simulink model "FOC_HF_G474"  (R2020b)
settings: Solver=FixedStepDiscrete  StartTime=0.0  StopTime=10  FixedStep=TsBSP  RelTol=1e-3
values from neighbouring files (symbols this model uses):
  BandwidthCurrentPI = 314.15926535897933    [G474_FOC_HF.sldd]
  Ld = 4.9E-5    [G474_FOC_HF.sldd]    (also in Hall_HFI_FOC_Data.sldd = 0.0004
  Ld_MODEL = 4.9E-5    [G474_FOC_HF.sldd]
  Lq = 4.9E-5    [G474_FOC_HF.sldd]    (also in Hall_HFI_FOC_Data.sldd = 0.00045
  Lq_MODEL = 4.9E-5    [G474_FOC_HF.sldd]
  MaxVoltage = 5.0    [G474_FOC_HF.sldd]
  PolePairs = 5.0    [G474_FOC_HF.sldd]
  PolePairs_MODEL = 5.0    [G474_FOC_HF.sldd]
  PWMHalfPeriod = 4199.0    [G474_FOC_HF.sldd]
  Rs = 0.082    [G474_FOC_HF.sldd]
  TsBSP = 2.0E-5    [G474_FOC_HF.sldd]
  TsFOC = 0.0001    [G474_FOC_HF.sldd]
  TsFOC_MODEL = 0.0001    [G474_FOC_HF.sldd]
undefined symbols (not defined in the file or in its folder): sigbuilder_block
libraries: pid_lib x4, mcbplantlib x1, autolibpmsminterior x1
(part 1 of 2)
PreSaveFcn:
  | cd(fileparts(which(bdroot)));
settings Model: DataDictionary=G474_FOC_HF.sldd  PacingRate=1000  Creator=beau_  LastModifiedBy=beau_
settings DataIOCC: SaveOutput=off  DSMLogging=off  SaveTime=off  ReturnWorkspaceOutputs=off
settings OptimizationCC: DefaultParameterBehavior=Inlined  EnhancedBackFolding=on  PassReuseOutputArgsAs=Individual arguments  ZeroExternalMemoryAtStartup=off  OptimizeBlockOrder=speed  DifferentSizesBufferReuse=on  OptimizationCustomize=off  EfficientTunableParamExpr=on
settings DebuggingCC: SignalRangeChecking=warning  ParameterPrecisionLossMsg=none  ParameterTunabilityLossMsg=error
settings HardwareCC: ProdBitPerPointer=32  ProdBitPerSizeT=32  ProdBitPerPtrDiffT=32  ProdLargestAtomicInteger=Long  ProdLargestAtomicFloat=Double  ProdWordSize=32  ProdHWDeviceType=ARM Compatible->ARM Cortex-M
settings SFSimCC: SimParseCustomCode=off  MATLABDynamicMemAlloc=off
settings RTWCC: Description=Embedded Coder  SystemTargetFile=ert.tlc  GenCodeOnly=on  TemplateMakefile=ert_default_tmf  RTWUseSimCustomCode=on
settings CodeAppCC: ForceParamTrailComments=on  GenerateComments=off  IgnoreCustomStorageClasses=off  OperatorAnnotations=on  SimulinkDataObjDesc=on  SFDataObjDesc=on  InsertBlockDesc=on
settings ERTTargetCC: TargetLangStandard=C99 (ISO)  CodeReplacementLibrary=ARM Cortex-M  GenerateSampleERTMain=on  SupportAbsoluteTime=off  SupportNonFinite=off  SupportComplex=off  InlinedParameterPlacement=NonHierarchical  ERTCustomFileTemplate=example_file_process.tlc

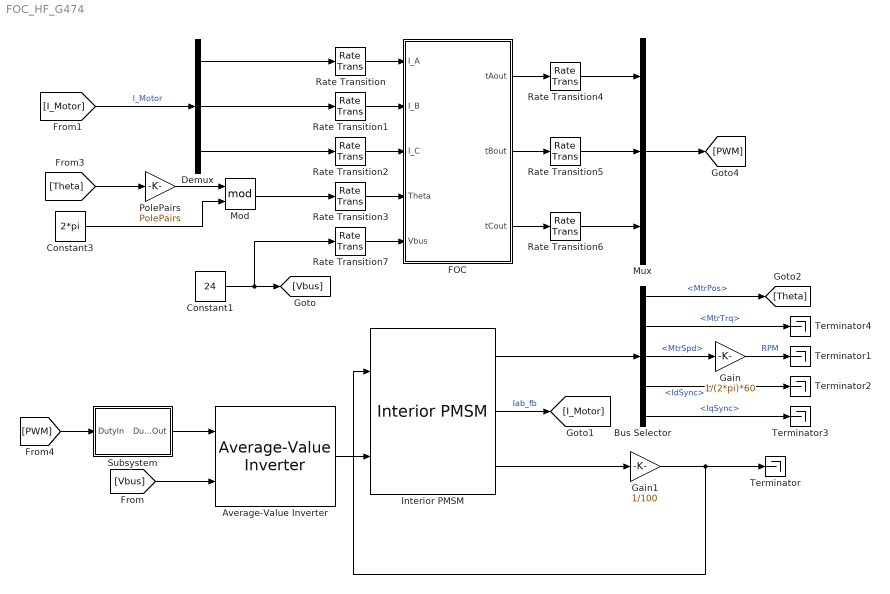
== system FOC_HF_G474 ==
  Average-Value Inverter : mcbplantlib/Average-Value Inverter
  Bus Selector : BusSelector  OutputSignals=MtrPos,MtrTrq,MtrSpd,IdSync,IqSync
  Constant1 : Constant  Value=24  SampleTime=TsBSP
  Constant3 : Constant  Value=2*pi  SampleTime=TsBSP
  Demux : Demux  Outputs=3
  FOC : Subsystem  SystemSampleTime=TsFOC
  Gain : Gain  Gain=1/(2*pi)*60
  Gain1 : Gain  Gain=1/100
  Interior PMSM : autolibpmsminterior/Interior PMSM  port_config=Torque  sim_type=Discrete  Ts=TsBSP  P=PolePairs_MODEL  Rs=Rs_MODEL  Ldq=[Ld_MODEL Lq_MODEL]  KConstText=Permanent flux linkage constant (lambda_pm):  lambda_pm=Flux_MODEL  Ke=159.9771  mechanical=[2.8e-4,1e-5,0.01]  idq0=[0 0]  theta_init=pi/4/PolePairs_MODEL  omega_init=0  KConst=Flux_MODEL  lambda_pm_calc=Flux_MODEL  Kt=0.07  RefBlkName='autolibpmsminterior/Interior PMSM'  aMode=5
      settings: SourceProductBaseCode=PW,MT,UV,VE,VP
  Mod : Math  Operator=mod  SaturateOnIntegerOverflow=on
  Mux : Mux  Inputs=3
  PolePairs : Gain  Gain=PolePairs
  Rate Transition{,1..3,7} (5 alike) : RateTransition
  Rate Transition4 : RateTransition  OutPortSampleTime=TsBSP
  Rate Transition5 : RateTransition  OutPortSampleTime=TsBSP
  Rate Transition6 : RateTransition  OutPortSampleTime=TsBSP
  Subsystem : Subsystem
  Terminator{,1..4} (5 alike) : Terminator
  wires:
  Average-Value Inverter/1 -> Interior PMSM/2
  Rate Transition4/1 -> Mux/1
  Interior PMSM/2 -> [I_Motor]  "Iab_fb"
  Rate Transition7/1 -> FOC/5(Vbus)
  Interior PMSM/3 -> Gain1/1
  Bus Selector/5 -> Terminator3/1  "<IqSync>"
  Bus Selector/4 -> Terminator2/1  "<IdSync>"
  [Vbus] -> Average-Value Inverter/2
  Mux/1 -> [PWM]
  Rate Transition2/1 -> FOC/3(I_C)
  Mod/1 -> Rate Transition3/1
  PolePairs/1 -> Mod/1
  Subsystem/1(DutyOut) -> Average-Value Inverter/1
  Constant1/1 -> Rate Transition7/1, [Vbus]
  Rate Transition3/1 -> FOC/4(Theta)
  Demux/3 -> Rate Transition2/1
  Rate Transition/1 -> FOC/1(I_A)
  Demux/1 -> Rate Transition/1
  Gain1/1 -> Interior PMSM/1, Terminator/1
  Rate Transition5/1 -> Mux/2
  Interior PMSM/1 -> Bus Selector/1
  Rate Transition6/1 -> Mux/3
  Bus Selector/1 -> [Theta]  "<MtrPos>"
  FOC/2(tBout) -> Rate Transition5/1
  [Theta] -> PolePairs/1
  FOC/3(tCout) -> Rate Transition6/1
  FOC/1(tAout) -> Rate Transition4/1
  Demux/2 -> Rate Transition1/1
  Bus Selector/3 -> Gain/1  "<MtrSpd>"
  Constant3/1 -> Mod/2
  Rate Transition1/1 -> FOC/2(I_B)
  [PWM] -> Subsystem/1(DutyIn)
  [I_Motor] -> Demux/1  "I_Motor"
  Gain/1 -> Terminator1/1  "RPM"
  Bus Selector/2 -> Terminator4/1  "<MtrTrq>"

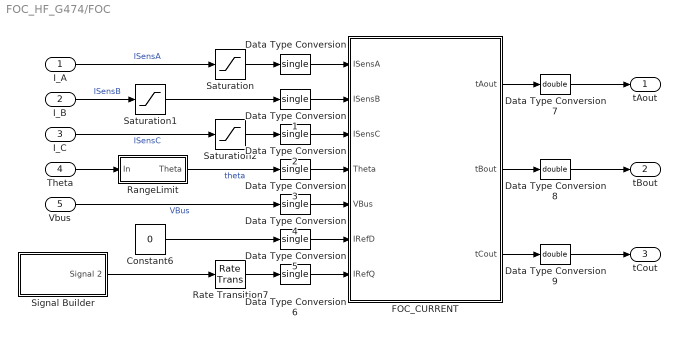
== system FOC_HF_G474/FOC ==
  I_A : Inport
  I_B : Inport  Port=2
  I_C : Inport  Port=3
  Theta : Inport  Port=4  OutMin=-2*pi  OutMax=2*pi
  Vbus : Inport  Port=5
  Constant6 : Constant  Value=0  SampleTime=-1
  Data Type Conversion{,1..6} (7 alike) : DataTypeConversion  OutDataTypeStr=single
  Data Type Conversion7 : DataTypeConversion  OutDataTypeStr=double
  Data Type Conversion8 : DataTypeConversion  OutDataTypeStr=double
  Data Type Conversion9 : DataTypeConversion  OutDataTypeStr=double
  FOC_CURRENT : Subsystem  TreatAsAtomicUnit=on  SystemSampleTime=TsFOC_MODEL
  RangeLimit : Subsystem
  Rate Transition7 : RateTransition
  Saturation : Saturate  UpperLimit=100  LowerLimit=-100
  Saturation1 : Saturate  UpperLimit=100  LowerLimit=-100
  Saturation2 : Saturate  UpperLimit=100  LowerLimit=-100
  Signal Builder : Subsystem  Tag=STV Subsys  LoadFcn=sigbuilder_block('load');  StartFcn=sigbuilder_block('start');  StopFcn=sigbuilder_block('stop');  ClipboardFcn=sigbuilder_block('clipboard');  mask(Sigbuilder block){tuvar=[0:10]}
      mask help: Simulink:masks:SigbuilderBlock_MD
      mask init:
      | if ~strcmp(get_param(bdroot(gcbh),'SimulationStatus'),'stopped') tuvar = sigbuilder_block('maskInit'); end
      settings: CopyFcn=sigbuilder_block('copy');  DeleteFcn=sigbuilder_block('delete');  ModelCloseFcn=sigbuilder_block('modelClose');  PreSaveFcn=sigbuilder_block('preSave');  PauseFcn=sigbuilder_block('pause');  ContinueFcn=sigbuilder_block('continue');  NameChangeFcn=sigbuilder_block('namechange');  OpenFcn=sigbuilder_block('open',[50.25 51 1141.5 581.25 ]);  CloseFcn=sigbuilder_block('close');
      mask Display: plot(0, 0, 100, 100,[2, 2, 32, 32, 2], [68, 8, 8, 68, 68],[32, 2], [38, 38], [32, 19, 2],[53, 60, 44], [32, 17, 17, 2],[16, 16, 31, 31]);txt = getActiveGroup(gcbh);text(2, 100, txt,'verticalAlignment', 'top');
  tAout : Outport
  tBout : Outport  Port=2
  tCout : Outport  Port=3
  wires:
  I_A/1 -> Saturation/1  "ISensA"
  I_C/1 -> Saturation2/1  "ISensC"
  Vbus/1 -> Data Type Conversion4/1  "VBus"
  I_B/1 -> Saturation1/1  "ISensB"
  Constant6/1 -> Data Type Conversion5/1
  Theta/1 -> RangeLimit/1(In)
  FOC_CURRENT/3(tCout) -> Data Type Conversion9/1
  FOC_CURRENT/1(tAout) -> Data Type Conversion7/1
  FOC_CURRENT/2(tBout) -> Data Type Conversion8/1
  Saturation/1 -> Data Type Conversion/1
  Saturation1/1 -> Data Type Conversion1/1
  Saturation2/1 -> Data Type Conversion2/1
  RangeLimit/1(Theta) -> Data Type Conversion3/1  "theta"
  Signal Builder/1(Signal 2) -> Rate Transition7/1
  Rate Transition7/1 -> Data Type Conversion6/1
  Data Type Conversion/1 -> FOC_CURRENT/1(ISensA)
  Data Type Conversion1/1 -> FOC_CURRENT/2(ISensB)
  Data Type Conversion2/1 -> FOC_CURRENT/3(ISensC)
  Data Type Conversion3/1 -> FOC_CURRENT/4(Theta)
  Data Type Conversion4/1 -> FOC_CURRENT/5(VBus)
  Data Type Conversion5/1 -> FOC_CURRENT/6(IRefD)
  Data Type Conversion6/1 -> FOC_CURRENT/7(IRefQ)
  Data Type Conversion7/1 -> tAout/1
  Data Type Conversion8/1 -> tBout/1
  Data Type Conversion9/1 -> tCout/1

== system FOC_HF_G474/Subsystem ==
  DutyIn : Inport
  Constant : Constant  Value=0.5  SampleTime=TsBSP
  Gain : Gain  Gain=1/PWMHalfPeriod  ParamDataTypeStr=single
  Gain1 : Gain  Gain=-1
  Sum : Sum  Inputs=|+-
  Sum1 : Sum  Inputs=|++
  DutyOut : Outport
  wires:
  Sum/1 -> Gain1/1
  Constant/1 -> Sum1/2, Sum/2
  DutyIn/1 -> Gain/1
  Gain1/1 -> Sum1/1
  Sum1/1 -> DutyOut/1
  Gain/1 -> Sum/1

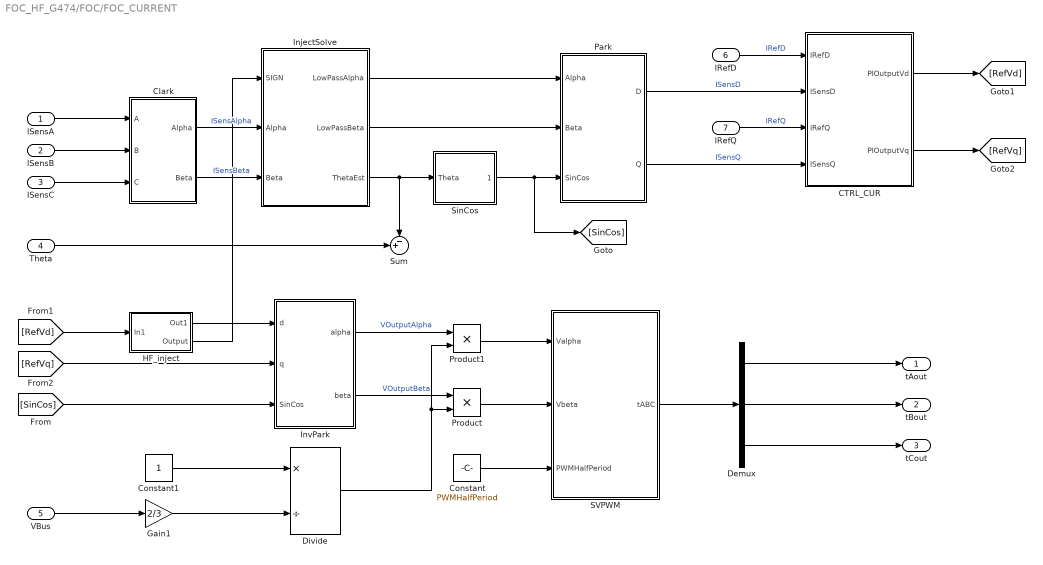
== system FOC_HF_G474/FOC/FOC_CURRENT ==
  ISensA : Inport  OutMin=-100  OutMax=100
  ISensB : Inport  Port=2  OutMin=-100  OutMax=100
  ISensC : Inport  Port=3  OutMin=-100  OutMax=100
  Theta : Inport  Port=4  OutMin=-2*pi  OutMax=2*pi
  VBus : Inport  Port=5  OutMin=0  OutMax=500
  IRefD : Inport  Port=6  OutMin=-50  OutMax=50
  IRefQ : Inport  Port=7  OutMin=-50  OutMax=50
  CTRL_CUR : Subsystem  TreatAsAtomicUnit=on
  Clark : Subsystem  TreatAsAtomicUnit=on
      settings: RTWSystemCode=Inline  RTWFcnNameOpts=Use subsystem name
      mask Display:
      | port_label('input',1,'a','texmode','on');
      | port_label('input',2,'b','texmode','on');
      | port_label('input',3,'c','texmode','on');
      | 
      | port_label('output',1,'\alpha','texmode','on');
      | port_label('output',2,'\beta','texmode','on');
      | 
      | fprintf('Clark');
  Constant : Constant  Value=PWMHalfPeriod  OutDataTypeStr=single  SampleTime=-1
  Constant1 : Constant  OutDataTypeStr=single  SampleTime=-1
  Demux : Demux  Outputs=3
  Divide : Product  Inputs=*/
  Gain1 : Gain  Gain=2/3
  HF_inject : Subsystem
  InjectSolve : Subsystem  TreatAsAtomicUnit=on
  InvPark : Subsystem  TreatAsAtomicUnit=on
      settings: RTWFcnNameOpts=Use subsystem name
      mask Display:
      | port_label('input',1,'d','texmode','on');
      | port_label('input',2,'q','texmode','on');
      | port_label('input',3,'\theta','texmode','on');
      | 
      | port_label('output',1,'\alpha','texmode','on');
      | port_label('output',2,'\beta','texmode','on');
      | 
      | fprintf('Inverse\nPark')
  Park : Subsystem  TreatAsAtomicUnit=on
      settings: RTWFcnNameOpts=Use subsystem name
      mask Display:
      | port_label('input',1,'\alpha','texmode','on');
      | port_label('input',2, '\beta','texmode','on');
      | port_label('input',3, 'sin\thetacos\theta','texmode','on');
      | 
      | port_label('output',1,'d','texmode','on');
      | port_label('output',2,'q','texmode','on');
      | fprintf('Park');
  Product : Product
  Product1 : Product
  SVPWM : Subsystem  TreatAsAtomicUnit=on
  SinCos : Subsystem
  Sum : Sum  Inputs=-+|
  tAout : Outport
  tBout : Outport  Port=2
  tCout : Outport  Port=3
  wires:
  Constant1/1 -> Divide/1
  CTRL_CUR/2(PIOutputVq) -> [RefVq]
  [RefVq] -> InvPark/2(q)
  InvPark/1(alpha) -> Product1/1  "VOutputAlpha"
  ISensB/1 -> Clark/2(B)
  IRefQ/1 -> CTRL_CUR/3(IRefQ)  "IRefQ"
  Divide/1 -> Product1/2, Product/2
  Product/1 -> SVPWM/2(Vbeta)
  Park/2(Q) -> CTRL_CUR/4(ISensQ)  "ISensQ"
  Gain1/1 -> Divide/2
  [SinCos] -> InvPark/3(SinCos)
  IRefD/1 -> CTRL_CUR/1(IRefD)  "IRefD"
  InvPark/2(beta) -> Product/1  "VOutputBeta"
  [RefVd] -> HF_inject/1(In1)
  Constant/1 -> SVPWM/3(PWMHalfPeriod)
  Park/1(D) -> CTRL_CUR/2(ISensD)  "ISensD"
  VBus/1 -> Gain1/1
  CTRL_CUR/1(PIOutputVd) -> [RefVd]
  SinCos/1(SinCos) -> [SinCos], Park/3(SinCos)
  ISensC/1 -> Clark/3(C)
  ISensA/1 -> Clark/1(A)
  Product1/1 -> SVPWM/1(Valpha)
  SVPWM/1(tABC) -> Demux/1
  Demux/1 -> tAout/1
  Demux/2 -> tBout/1
  Demux/3 -> tCout/1
  HF_inject/1(Out1) -> InvPark/1(d)
  Clark/1(Alpha) -> InjectSolve/2(Alpha)  "ISensAlpha"
  Clark/2(Beta) -> InjectSolve/3(Beta)  "ISensBeta"
  HF_inject/2(Output) -> InjectSolve/1(SIGN)
  InjectSolve/1(LowPassAlpha) -> Park/1(Alpha)
  InjectSolve/2(LowPassBeta) -> Park/2(Beta)
  InjectSolve/3(ThetaEst) -> Sum/1, SinCos/1(Theta)
  Theta/1 -> Sum/2

== system FOC_HF_G474/FOC/RangeLimit ==
  In : Inport
  Constant : Constant  Value=pi  SampleTime=-1
  Constant1 : Constant  Value=-pi  SampleTime=-1
  If : If  NumInputs=2  IfExpression=u1  ElseIfExpressions=u2
  If Action Subsystem : Subsystem  TreatAsAtomicUnit=on
  If Action Subsystem1 : Subsystem  TreatAsAtomicUnit=on
  If Action Subsystem2 : Subsystem  TreatAsAtomicUnit=on
  Merge : Merge  Inputs=3
  Relational Operator : RelationalOperator  Operator=>  OutDataTypeStr=boolean  RndMeth=Simplest
  Relational Operator1 : RelationalOperator  Operator=<  OutDataTypeStr=boolean  RndMeth=Simplest
  Theta : Outport  OutMin=-pi  OutMax=pi
  wires:
  Relational Operator/1 -> If/1
  Constant/1 -> Relational Operator/2
  Constant1/1 -> Relational Operator1/2
  In/1 -> Relational Operator1/1, If Action Subsystem2/1(In1), If Action Subsystem1/1(In1), If Action Subsystem/1(In1), Relational Operator/1
  Relational Operator1/1 -> If/2
  Merge/1 -> Theta/1
  If/3 -> If Action Subsystem2/Action
  If/2 -> If Action Subsystem/Action
  If/1 -> If Action Subsystem1/Action
  If Action Subsystem2/1(Out1) -> Merge/1
  If Action Subsystem/1(Out1) -> Merge/2
  If Action Subsystem1/1(Out1) -> Merge/3

== system FOC_HF_G474/FOC/Signal Builder ==
  Demux : Demux  Tag=STV Demux  Outputs=1
      settings: DisplayOption=none
  FromWs : FromWorkspace  Tag=STV FromWs  VariableName=tuvar
      SigBuilderData=|
      | common.afterFinalStr = 'Extrapolate'
      | common.sampleTime = 0
      | dataSet.timeRange = [0 10]
      | dataSet.name = 'Group 1'
      | sbobj.Groups.Name = 'Group 1'
      | sbobj.Groups.Signals.Name = 'Signal 2'
      | sbobj.Groups.Signals.XData = [0 0.53 0.53 0.99 0.99 1.98 1.98 3 4 4 5.01 5.01 6 6 7 7.99 7.99 9 9 10]
      | sbobj.Groups.Signals.YData = [0 0 0.9 0.9 0.85 2.15 2.25 2.35 -2.3 -2.4 -2.4 -2.5 -2.5 0.8 0.8 0.8 1.6 1.6 2 2]
  Signal 2 : Outport  Tag=STV Outport
  wires:
  FromWs/1 -> Demux/1
  Demux/1 -> Signal 2/1

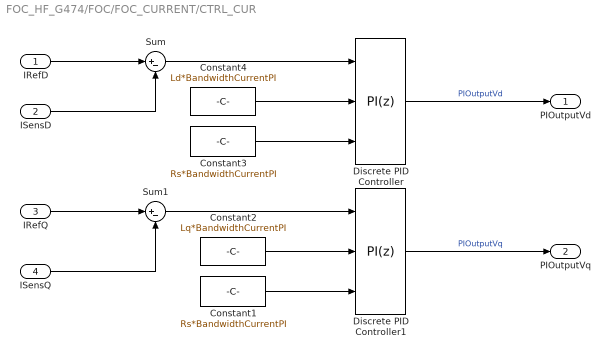
== system FOC_HF_G474/FOC/FOC_CURRENT/CTRL_CUR ==
  IRefD : Inport
  ISensD : Inport  Port=2
  IRefQ : Inport  Port=3
  ISensQ : Inport  Port=4
  Constant1 : Constant  Value=Rs*BandwidthCurrentPI  OutDataTypeStr=single  SampleTime=-1
  Constant2 : Constant  Value=Lq*BandwidthCurrentPI  OutDataTypeStr=single  SampleTime=-1
  Constant3 : Constant  Value=Rs*BandwidthCurrentPI  OutDataTypeStr=single  SampleTime=-1
  Constant4 : Constant  Value=Ld*BandwidthCurrentPI  OutDataTypeStr=single  SampleTime=-1
  Discrete PID Controller : pid_lib/PID Controller  Controller=PI  Form=Parallel  TimeDomain=Discrete-time  UseExternalTs=off  SampleTime=-1  IntegratorMethod=Forward Euler  FilterMethod=Forward Euler  ControllerParametersSource=external  P=1  I=1  D=0  UseFilter=off  N=100  TunerSelectOption=Transfer Function Based (PID Tuner App)  ZeroCross=off  InitialConditionSource=internal  InitialConditionForIntegrator=0  InitialConditionForFilter=0  DifferentiatorICPrevScaledInput=0  ExternalReset=none  TrackingMode=off  Kt=1  LimitOutput=on  SatLimitsSource=internal  UpperSaturationLimit=MaxVoltage  LowerSaturationLimit=-MaxVoltage  LinearizeAsGain=off  AntiWindupMode=clamping  Kb=1  POutMin=[]  POutMax=[]  IOutMin=[]  IOutMax=[]  DOutMin=[]  DOutMax=[]  NOutMin=[]  NOutMax=[]  SumOutMin=[]  SumOutMax=[]  SaturationOutDataTypeStr=Inherit: Inherit via back propagation  SaturationOutMin=[]  SaturationOutMax=[]  PParamMin=[]  PParamMax=[]  IParamMin=[]  IParamMax=[]  DParamMin=[]  DParamMax=[]  NParamMin=[]  NParamMax=[]  KbParamMin=[]  KbParamMax=[]  KtParamMin=[]  KtParamMax=[]  KbOutMin=[]  KbOutMax=[]  KtOutMin=[]  KtOutMax=[]  IntegratorOutMin=[]  IntegratorOutMax=[]  FilterOutMin=[]  FilterOutMax=[]  SumI1OutMin=[]  SumI1OutMax=[]  SumI2OutMin=[]  SumI2OutMax=[]  SumI3OutMin=[]  SumI3OutMax=[]  SumI4OutMin=[]  SumI4OutMax=[]  SumDOutMin=[]  SumDOutMax=[]  DifferentiatorOutMin=[]  DifferentiatorOutMax=[]  FilterDiffOutCoefMin=[]  FilterDiffOutCoefMax=[]  ReciprocalOutMin=[]  ReciprocalOutMax=[]  SumDenOutMin=[]  SumDenOutMax=[]  SumNumOutMin=[]  SumNumOutMax=[]  DivideOutMin=[]  DivideOutMax=[]  UdiffTsProdOutMin=[]  UdiffTsProdOutMax=[]  NTsProdOutMin=[]  NTsProdOutMax=[]  UintegralTsProdOutMin=[]  UintegralTsProdOutMax=[]  UngainTsProdOutMin=[]  UngainTsProdOutMax=[]  IntegratorContinuousStateAttributes=''  IntegratorStateMustResolveToSignalObject=off  IntegratorRTWStateStorageClass=Auto  FilterContinuousStateAttributes=''  FilterStateMustResolveToSignalObject=off  FilterRTWStateStorageClass=Auto  ParallelPVariant=ExternalParameters  IdealPVariant=Disabled  IVariant=ExternalParameters  DVariant=Disabled  IntegratorVariant=Discrete  SatVariant=Enabled  AWVariant=DiscClampingParallel  PCopyVariant=Disabled  TRVariant=Disabled  FdbkBlocksVariant=Forward  IdealPFdbkVariant=Disabled  SatFdbkVariant=Disabled  DerivativeFilterVariant=Disabled  NVariant=Disabled  NCopyVariant=Disabled_SignalSpec  FilterICVariant=Disabled  IntegratorICVariant=InternalICs  ExternalResetVariant=Disabled  TRSumVariant=Passthrough  SumFdbkVariant=Disabled  SumVariant=Sum_PI  TsampFilterVariant=InternalTs  TsampNgainVariant=Passthrough  TsampIntegralVariant=Passthrough  ExternalSaturationOutDataTypeStr=Inherit: Same as second input
  Discrete PID Controller1 : pid_lib/PID Controller  Controller=PI  Form=Parallel  TimeDomain=Discrete-time  UseExternalTs=off  SampleTime=-1  IntegratorMethod=Forward Euler  FilterMethod=Forward Euler  ControllerParametersSource=external  P=1  I=1  D=0  UseFilter=off  N=100  TunerSelectOption=Transfer Function Based (PID Tuner App)  ZeroCross=off  InitialConditionSource=internal  InitialConditionForIntegrator=0  InitialConditionForFilter=0  DifferentiatorICPrevScaledInput=0  ExternalReset=none  TrackingMode=off  Kt=1  LimitOutput=on  SatLimitsSource=internal  UpperSaturationLimit=MaxVoltage  LowerSaturationLimit=-MaxVoltage  LinearizeAsGain=off  AntiWindupMode=clamping  Kb=1  POutMin=[]  POutMax=[]  IOutMin=[]  IOutMax=[]  DOutMin=[]  DOutMax=[]  NOutMin=[]  NOutMax=[]  SumOutMin=[]  SumOutMax=[]  SaturationOutDataTypeStr=Inherit: Inherit via back propagation  SaturationOutMin=[]  SaturationOutMax=[]  PParamMin=[]  PParamMax=[]  IParamMin=[]  IParamMax=[]  DParamMin=[]  DParamMax=[]  NParamMin=[]  NParamMax=[]  KbParamMin=[]  KbParamMax=[]  KtParamMin=[]  KtParamMax=[]  KbOutMin=[]  KbOutMax=[]  KtOutMin=[]  KtOutMax=[]  IntegratorOutMin=[]  IntegratorOutMax=[]  FilterOutMin=[]  FilterOutMax=[]  SumI1OutMin=[]  SumI1OutMax=[]  SumI2OutMin=[]  SumI2OutMax=[]  SumI3OutMin=[]  SumI3OutMax=[]  SumI4OutMin=[]  SumI4OutMax=[]  SumDOutMin=[]  SumDOutMax=[]  DifferentiatorOutMin=[]  DifferentiatorOutMax=[]  FilterDiffOutCoefMin=[]  FilterDiffOutCoefMax=[]  ReciprocalOutMin=[]  ReciprocalOutMax=[]  SumDenOutMin=[]  SumDenOutMax=[]  SumNumOutMin=[]  SumNumOutMax=[]  DivideOutMin=[]  DivideOutMax=[]  UdiffTsProdOutMin=[]  UdiffTsProdOutMax=[]  NTsProdOutMin=[]  NTsProdOutMax=[]  UintegralTsProdOutMin=[]  UintegralTsProdOutMax=[]  UngainTsProdOutMin=[]  UngainTsProdOutMax=[]  IntegratorContinuousStateAttributes=''  IntegratorStateMustResolveToSignalObject=off  IntegratorRTWStateStorageClass=Auto  FilterContinuousStateAttributes=''  FilterStateMustResolveToSignalObject=off  FilterRTWStateStorageClass=Auto  ParallelPVariant=ExternalParameters  IdealPVariant=Disabled  IVariant=ExternalParameters  DVariant=Disabled  IntegratorVariant=Discrete  SatVariant=Enabled  AWVariant=DiscClampingParallel  PCopyVariant=Disabled  TRVariant=Disabled  FdbkBlocksVariant=Forward  IdealPFdbkVariant=Disabled  SatFdbkVariant=Disabled  DerivativeFilterVariant=Disabled  NVariant=Disabled  NCopyVariant=Disabled_SignalSpec  FilterICVariant=Disabled  IntegratorICVariant=InternalICs  ExternalResetVariant=Disabled  TRSumVariant=Passthrough  SumFdbkVariant=Disabled  SumVariant=Sum_PI  TsampFilterVariant=InternalTs  TsampNgainVariant=Passthrough  TsampIntegralVariant=Passthrough  ExternalSaturationOutDataTypeStr=Inherit: Same as second input
  Sum : Sum  Inputs=|+-
  Sum1 : Sum  Inputs=|+-
  PIOutputVd : Outport
  PIOutputVq : Outport  Port=2
  wires:
  IRefD/1 -> Sum/1
  Sum/1 -> Discrete PID Controller/1
  Discrete PID Controller/1 -> PIOutputVd/1  "PIOutputVd"
  ISensD/1 -> Sum/2
  Constant4/1 -> Discrete PID Controller/2
  Constant3/1 -> Discrete PID Controller/3
  IRefQ/1 -> Sum1/1
  Constant2/1 -> Discrete PID Controller1/2
  Sum1/1 -> Discrete PID Controller1/1
  ISensQ/1 -> Sum1/2
  Constant1/1 -> Discrete PID Controller1/3
  Discrete PID Controller1/1 -> PIOutputVq/1  "PIOutputVq"

== system FOC_HF_G474/FOC/FOC_CURRENT/Clark ==
  A : Inport
  B : Inport  Port=2
  C : Inport  Port=3
  Gain : Gain  Gain=single(2/3)
  Gain1 : Gain  Gain=0.5
  Gain2 : Gain  Gain=single(sqrt(3)/3)
  Sum : Sum  Inputs=|++
  Sum1 : Sum  Inputs=|+-
  Sum2 : Sum  Inputs=+-|
  Alpha : Outport
  Beta : Outport  Port=2
  wires:
  Sum/1 -> Gain1/1
  Gain2/1 -> Beta/1
  B/1 -> Sum2/1, Sum/1
  Gain1/1 -> Sum1/2
  Gain/1 -> Alpha/1
  Sum2/1 -> Gain2/1
  C/1 -> Sum2/2, Sum/2
  A/1 -> Sum1/1
  Sum1/1 -> Gain/1

== system FOC_HF_G474/FOC/FOC_CURRENT/HF_inject ==
  In1 : Inport
  Gain : Gain  Gain=-1  OutDataTypeStr=single
  Gain1 : Gain  Gain=2
  Sum : Sum  Inputs=|++
  Unit Delay : UnitDelay  InitialCondition=1  SampleTime=-1  HasFrameUpgradeWarning=on
  Out1 : Outport
  Output : Outport  Port=2
  wires:
  In1/1 -> Sum/1
  Sum/1 -> Out1/1
  Unit Delay/1 -> Gain/1
  Gain/1 -> Unit Delay/1, Gain1/1
  Gain1/1 -> Output/1, Sum/2

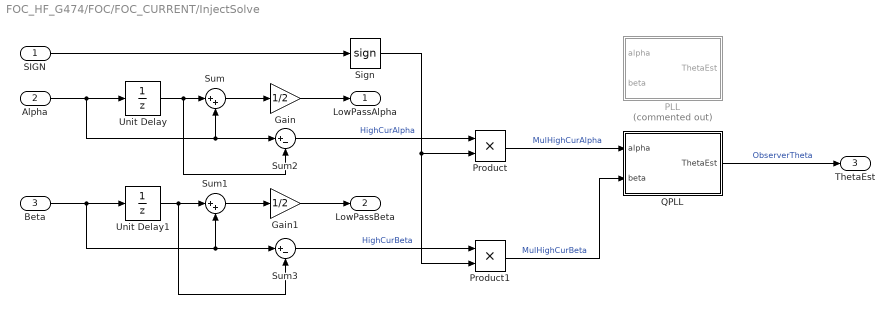
== system FOC_HF_G474/FOC/FOC_CURRENT/InjectSolve ==
  SIGN : Inport
  Alpha : Inport  Port=2
  Beta : Inport  Port=3
  Gain : Gain  Gain=1/2
  Gain1 : Gain  Gain=1/2
  PLL : Subsystem  Commented=on
  Product : Product
  Product1 : Product
  QPLL : Subsystem
  Sign : Signum
  Sum : Sum  Inputs=|++
  Sum1 : Sum  Inputs=|++
  Sum2 : Sum  Inputs=|+-
  Sum3 : Sum  Inputs=|+-
  Unit Delay : UnitDelay  SampleTime=-1  HasFrameUpgradeWarning=on
  Unit Delay1 : UnitDelay  SampleTime=-1  HasFrameUpgradeWarning=on
  LowPassAlpha : Outport
  LowPassBeta : Outport  Port=2
  ThetaEst : Outport  Port=3  InitialOutput=[0]
  wires:
  Alpha/1 -> Unit Delay/1, Sum/2, Sum2/1
  Unit Delay/1 -> Sum2/2, Sum/1
  Sum/1 -> Gain/1
  Gain/1 -> LowPassAlpha/1
  Sum1/1 -> Gain1/1
  Unit Delay1/1 -> Sum3/2, Sum1/1
  Beta/1 -> Unit Delay1/1, Sum1/2, Sum3/1
  Gain1/1 -> LowPassBeta/1
  Sum2/1 -> Product/1  "HighCurAlpha"
  Sign/1 -> Product/2, Product1/2
  Sum3/1 -> Product1/1  "HighCurBeta"
  Product/1 -> QPLL/1(alpha)  "MulHighCurAlpha"
  Product1/1 -> QPLL/2(beta)  "MulHighCurBeta"
  QPLL/1(ThetaEst) -> ThetaEst/1  "ObserverTheta"
  SIGN/1 -> Sign/1

== system FOC_HF_G474/FOC/FOC_CURRENT/InvPark ==
  d : Inport
  q : Inport  Port=2
  SinCos : Inport  Port=3
  Demux : Demux  Outputs=2
  Product{,1..3} (4 alike) : Product
  Sum : Sum  Inputs=|+-
  Sum1 : Sum  Inputs=|++
  alpha : Outport
  beta : Outport  Port=2
  wires:
  Sum/1 -> alpha/1
  SinCos/1 -> Demux/1
  d/1 -> Product2/1, Product/1
  Demux/2 -> Product/2, Product3/2
  q/1 -> Product3/1, Product1/1
  Demux/1 -> Product1/2, Product2/2
  Product/1 -> Sum/1
  Product1/1 -> Sum/2
  Product2/1 -> Sum1/1
  Product3/1 -> Sum1/2
  Sum1/1 -> beta/1

== system FOC_HF_G474/FOC/FOC_CURRENT/Park ==
  Alpha : Inport
  Beta : Inport  Port=2
  SinCos : Inport  Port=3
  Demux : Demux  Outputs=2
  Product{,1..3} (4 alike) : Product
  Sum : Sum  Inputs=|++
  Sum1 : Sum  Inputs=|-+
  D : Outport
  Q : Outport  Port=2
  wires:
  Beta/1 -> Product3/1, Product1/1
  Alpha/1 -> Product2/1, Product/1
  SinCos/1 -> Demux/1
  Demux/2 -> Product/2, Product3/2
  Demux/1 -> Product1/2, Product2/2
  Product/1 -> Sum/1
  Product1/1 -> Sum/2
  Sum/1 -> D/1
  Product2/1 -> Sum1/1
  Product3/1 -> Sum1/2
  Sum1/1 -> Q/1

== system FOC_HF_G474/FOC/FOC_CURRENT/SVPWM ==
  Valpha : Inport
  Vbeta : Inport  Port=2
  PWMHalfPeriod : Inport  Port=3
  CalcPWM : Subsystem
  JudgeSector : Subsystem
  tABC : Outport
  wires:
  CalcPWM/1(tABC) -> tABC/1
  Vbeta/1 -> CalcPWM/2(Vbeta), JudgeSector/2(Vbeta)
  JudgeSector/1(Sector) -> CalcPWM/3(Sector)
  Valpha/1 -> JudgeSector/1(Valpha), CalcPWM/1(Valpha)
  PWMHalfPeriod/1 -> CalcPWM/4(PWMHalfPeriod)

== system FOC_HF_G474/FOC/FOC_CURRENT/SinCos ==
  Theta : Inport
  Mux : Mux  Inputs=2
  Sin : Trigonometry  Operator=sincos
  SinCos : Outport
  wires:
  Theta/1 -> Sin/1
  Mux/1 -> SinCos/1
  Sin/2 -> Mux/2
  Sin/1 -> Mux/1

== system FOC_HF_G474/FOC/RangeLimit/If Action Subsystem ==
  In1 : Inport
  Action Port : ActionPort  ActionPortLabel=elseif(u2)
  Constant : Constant  Value=2*pi  SampleTime=-1
  Sum : Sum  Inputs=|++
  Out1 : Outport
  wires:
  In1/1 -> Sum/1
  Constant/1 -> Sum/2
  Sum/1 -> Out1/1

== system FOC_HF_G474/FOC/RangeLimit/If Action Subsystem1 ==
  In1 : Inport
  Action Port : ActionPort  ActionPortLabel=if(u1)
  Constant : Constant  Value=2*pi  SampleTime=-1
  Sum : Sum  Inputs=|+-
  Out1 : Outport
  wires:
  In1/1 -> Sum/1
  Constant/1 -> Sum/2
  Sum/1 -> Out1/1

== system FOC_HF_G474/FOC/RangeLimit/If Action Subsystem2 ==
  In1 : Inport
  Action Port : ActionPort  ActionPortLabel=else
  Out1 : Outport
  wires:
  In1/1 -> Out1/1

== system FOC_HF_G474/FOC/FOC_CURRENT/InjectSolve/PLL ==
  alpha : Inport
  beta : Inport  Port=2
  Atan2 : Trigonometry  Operator=atan2
  PID Controller : pid_lib/PID Controller  Controller=PI  Form=Parallel  TimeDomain=Discrete-time  UseExternalTs=off  SampleTime=-1  IntegratorMethod=Forward Euler  FilterMethod=Forward Euler  ControllerParametersSource=internal  P=6e3  I=8e4  D=0.000000000000000  UseFilter=on  N=99.750416146353601  TunerSelectOption=Transfer Function Based (PID Tuner App)  ZeroCross=off  InitialConditionSource=internal  InitialConditionForIntegrator=0  InitialConditionForFilter=0  DifferentiatorICPrevScaledInput=0  ExternalReset=none  TrackingMode=off  Kt=1  LimitOutput=off  SatLimitsSource=internal  UpperSaturationLimit=pi/2  LowerSaturationLimit=-pi/2  LinearizeAsGain=on  AntiWindupMode=none  Kb=1  POutMin=[]  POutMax=[]  IOutMin=[]  IOutMax=[]  DOutMin=[]  DOutMax=[]  NOutMin=[]  NOutMax=[]  SumOutMin=[]  SumOutMax=[]  SaturationOutMin=[]  SaturationOutMax=[]  PParamMin=[]  PParamMax=[]  IParamMin=[]  IParamMax=[]  DParamMin=[]  DParamMax=[]  NParamMin=[]  NParamMax=[]  KbParamMin=[]  KbParamMax=[]  KtParamMin=[]  KtParamMax=[]  KbOutMin=[]  KbOutMax=[]  KtOutMin=[]  KtOutMax=[]  IntegratorOutMin=[]  IntegratorOutMax=[]  FilterOutMin=[]  FilterOutMax=[]  SumI1OutMin=[]  SumI1OutMax=[]  SumI2OutMin=[]  SumI2OutMax=[]  SumI3OutMin=[]  SumI3OutMax=[]  SumI4OutMin=[]  SumI4OutMax=[]  SumDOutMin=[]  SumDOutMax=[]  DifferentiatorOutMin=[]  DifferentiatorOutMax=[]  FilterDiffOutCoefMin=[]  FilterDiffOutCoefMax=[]  ReciprocalOutMin=[]  ReciprocalOutMax=[]  SumDenOutMin=[]  SumDenOutMax=[]  SumNumOutMin=[]  SumNumOutMax=[]  DivideOutMin=[]  DivideOutMax=[]  UdiffTsProdOutMin=[]  UdiffTsProdOutMax=[]  NTsProdOutMin=[]  NTsProdOutMax=[]  UintegralTsProdOutMin=[]  UintegralTsProdOutMax=[]  UngainTsProdOutMin=[]  UngainTsProdOutMax=[]  IntegratorContinuousStateAttributes=''  IntegratorStateMustResolveToSignalObject=off  IntegratorRTWStateStorageClass=Auto  FilterContinuousStateAttributes=''  FilterStateMustResolveToSignalObject=off  FilterRTWStateStorageClass=Auto  ParallelPVariant=InternalParameters  IdealPVariant=Disabled  IVariant=InternalParameters  DVariant=Disabled  IntegratorVariant=Discrete  SatVariant=Disabled  AWVariant=Passthrough  PCopyVariant=Disabled  TRVariant=Disabled  FdbkBlocksVariant=Forward  IdealPFdbkVariant=Disabled  SatFdbkVariant=Disabled  DerivativeFilterVariant=Disabled  NVariant=Disabled  NCopyVariant=Disabled_SignalSpec  FilterICVariant=Disabled  IntegratorICVariant=InternalICs  ExternalResetVariant=Disabled  TRSumVariant=Passthrough  SumFdbkVariant=Disabled  SumVariant=Sum_PI  TsampFilterVariant=InternalTs  TsampNgainVariant=Passthrough  TsampIntegralVariant=Passthrough  ExternalSaturationOutDataTypeStr=Inherit: Same as second input
  SpeedToTheta : Subsystem
  Subsystem : Subsystem
  Sum5 : Sum  Inputs=|+-
  ThetaEst : Outport
  wires:
  SpeedToTheta/1(Out1) -> ThetaEst/1, Sum5/2  "ThetaEst1"
  Sum5/1 -> Subsystem/1(In1)
  PID Controller/1 -> SpeedToTheta/1(In1)
  Atan2/1 -> Sum5/1
  Subsystem/1(Output) -> PID Controller/1
  alpha/1 -> Atan2/2
  beta/1 -> Atan2/1

== system FOC_HF_G474/FOC/FOC_CURRENT/InjectSolve/QPLL ==
  alpha : Inport
  beta : Inport  Port=2
  Cos : Trigonometry  Operator=cos
  PIDTheta_Ctrl1 : pid_lib/PID Controller  Controller=PI  Form=Parallel  TimeDomain=Discrete-time  UseExternalTs=off  SampleTime=-1  IntegratorMethod=Forward Euler  FilterMethod=Forward Euler  ControllerParametersSource=internal  P=2*0.707*500  I=500*500  D=0  UseFilter=on  N=100  TunerSelectOption=Transfer Function Based (PID Tuner App)  ZeroCross=off  InitialConditionSource=internal  InitialConditionForIntegrator=0  InitialConditionForFilter=0  DifferentiatorICPrevScaledInput=0  ExternalReset=none  TrackingMode=off  Kt=1  LimitOutput=on  SatLimitsSource=internal  UpperSaturationLimit=2*pi*200  LowerSaturationLimit=-2*pi*200  LinearizeAsGain=off  AntiWindupMode=clamping  Kb=50  POutMin=[]  POutMax=[]  IOutMin=[]  IOutMax=[]  DOutMin=[]  DOutMax=[]  NOutMin=[]  NOutMax=[]  SumOutMin=[]  SumOutMax=[]  SaturationOutDataTypeStr=Inherit: Inherit via back propagation  SaturationOutMin=[]  SaturationOutMax=[]  PParamMin=[]  PParamMax=[]  IParamMin=[]  IParamMax=[]  DParamMin=[]  DParamMax=[]  NParamMin=[]  NParamMax=[]  KbParamMin=[]  KbParamMax=[]  KtParamMin=[]  KtParamMax=[]  KbOutMin=[]  KbOutMax=[]  KtOutMin=[]  KtOutMax=[]  IntegratorOutMin=[]  IntegratorOutMax=[]  FilterOutMin=[]  FilterOutMax=[]  SumI1OutMin=[]  SumI1OutMax=[]  SumI2OutMin=[]  SumI2OutMax=[]  SumI3OutMin=[]  SumI3OutMax=[]  SumI4OutMin=[]  SumI4OutMax=[]  SumDOutMin=[]  SumDOutMax=[]  DifferentiatorOutMin=[]  DifferentiatorOutMax=[]  FilterDiffOutCoefMin=[]  FilterDiffOutCoefMax=[]  ReciprocalOutMin=[]  ReciprocalOutMax=[]  SumDenOutMin=[]  SumDenOutMax=[]  SumNumOutMin=[]  SumNumOutMax=[]  DivideOutMin=[]  DivideOutMax=[]  UdiffTsProdOutMin=[]  UdiffTsProdOutMax=[]  NTsProdOutMin=[]  NTsProdOutMax=[]  UintegralTsProdOutMin=[]  UintegralTsProdOutMax=[]  UngainTsProdOutMin=[]  UngainTsProdOutMax=[]  IntegratorContinuousStateAttributes=''  IntegratorStateMustResolveToSignalObject=off  IntegratorRTWStateStorageClass=Auto  FilterContinuousStateAttributes=''  FilterStateMustResolveToSignalObject=off  FilterRTWStateStorageClass=Auto  ParallelPVariant=InternalParameters  IdealPVariant=Disabled  IVariant=InternalParameters  DVariant=Disabled  IntegratorVariant=Discrete  SatVariant=Enabled  AWVariant=DiscClampingParallel  PCopyVariant=Disabled  TRVariant=Disabled  FdbkBlocksVariant=Forward  IdealPFdbkVariant=Disabled  SatFdbkVariant=Disabled  DerivativeFilterVariant=Disabled  NVariant=Disabled  NCopyVariant=Disabled_SignalSpec  FilterICVariant=Disabled  IntegratorICVariant=InternalICs  ExternalResetVariant=Disabled  TRSumVariant=Passthrough  SumFdbkVariant=Disabled  SumVariant=Sum_PI  TsampFilterVariant=InternalTs  TsampNgainVariant=Passthrough  TsampIntegralVariant=Passthrough  ExternalSaturationOutDataTypeStr=Inherit: Same as second input
  Product : Product
  Product1 : Product
  Sin : Trigonometry
  SpeedToTheta : Subsystem
  Sum5 : Sum  Inputs=|-+
  ThetaEst : Outport
  wires:
  Product1/1 -> Sum5/1
  alpha/1 -> Product1/1
  beta/1 -> Product/2
  Product/1 -> Sum5/2
  PIDTheta_Ctrl1/1 -> SpeedToTheta/1(In1)
  Sin/1 -> Product1/2
  Cos/1 -> Product/1
  Sum5/1 -> PIDTheta_Ctrl1/1
  [theta_hat] -> Cos/1, Sin/1
  SpeedToTheta/1(Out1) -> [theta_hat], ThetaEst/1

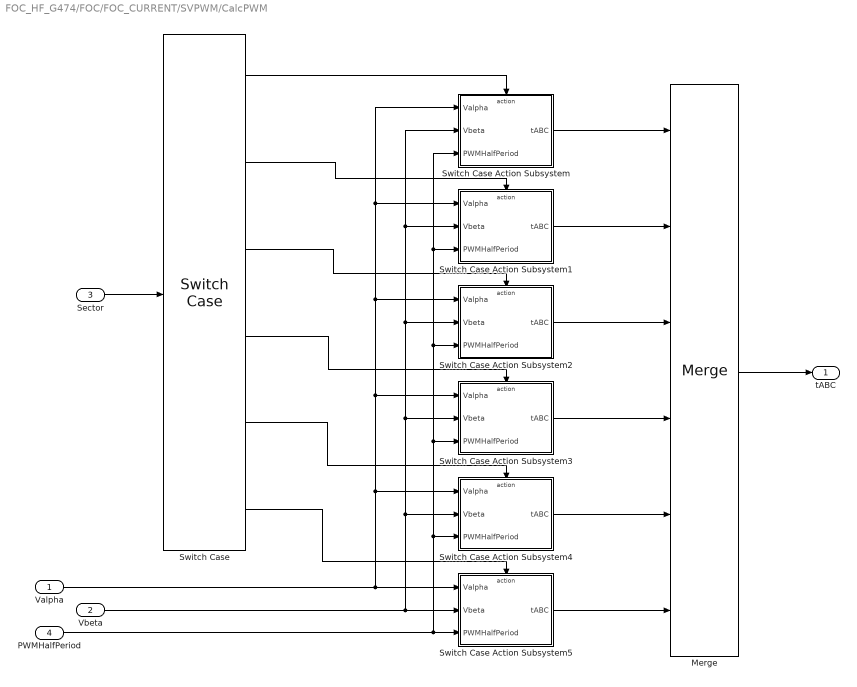
== system FOC_HF_G474/FOC/FOC_CURRENT/SVPWM/CalcPWM ==
  Valpha : Inport
  Vbeta : Inport  Port=2
  Sector : Inport  Port=3
  PWMHalfPeriod : Inport  Port=4
  Merge : Merge  Inputs=6  InitialOutput=[0 0 0]
  Switch Case : SwitchCase  CaseConditions={1,2,3,4,5,6}  ShowDefaultCase=off
  Switch Case Action Subsystem : Subsystem  TreatAsAtomicUnit=on
  Switch Case Action Subsystem1 : Subsystem  TreatAsAtomicUnit=on
  Switch Case Action Subsystem2 : Subsystem  TreatAsAtomicUnit=on
  Switch Case Action Subsystem3 : Subsystem  TreatAsAtomicUnit=on
  Switch Case Action Subsystem4 : Subsystem  TreatAsAtomicUnit=on
  Switch Case Action Subsystem5 : Subsystem  TreatAsAtomicUnit=on
  tABC : Outport
  wires:
  Sector/1 -> Switch Case/1
  Switch Case/1 -> Switch Case Action Subsystem/Action
  Switch Case/2 -> Switch Case Action Subsystem1/Action
  Switch Case/3 -> Switch Case Action Subsystem2/Action
  Switch Case/4 -> Switch Case Action Subsystem3/Action
  Switch Case/5 -> Switch Case Action Subsystem4/Action
  Switch Case/6 -> Switch Case Action Subsystem5/Action
  Valpha/1 -> Switch Case Action Subsystem/1(Valpha), Switch Case Action Subsystem1/1(Valpha), Switch Case Action Subsystem2/1(Valpha), Switch Case Action Subsystem3/1(Valpha), Switch Case Action Subsystem4/1(Valpha), Switch Case Action Subsystem5/1(Valpha)
  Vbeta/1 -> Switch Case Action Subsystem/2(Vbeta), Switch Case Action Subsystem1/2(Vbeta), Switch Case Action Subsystem2/2(Vbeta), Switch Case Action Subsystem3/2(Vbeta), Switch Case Action Subsystem4/2(Vbeta), Switch Case Action Subsystem5/2(Vbeta)
  PWMHalfPeriod/1 -> Switch Case Action Subsystem/3(PWMHalfPeriod), Switch Case Action Subsystem1/3(PWMHalfPeriod), Switch Case Action Subsystem2/3(PWMHalfPeriod), Switch Case Action Subsystem3/3(PWMHalfPeriod), Switch Case Action Subsystem4/3(PWMHalfPeriod), Switch Case Action Subsystem5/3(PWMHalfPeriod)
  Switch Case Action Subsystem/1(tABC) -> Merge/1
  Switch Case Action Subsystem1/1(tABC) -> Merge/2
  Switch Case Action Subsystem2/1(tABC) -> Merge/3
  Switch Case Action Subsystem3/1(tABC) -> Merge/4
  Switch Case Action Subsystem4/1(tABC) -> Merge/5
  Switch Case Action Subsystem5/1(tABC) -> Merge/6
  Merge/1 -> tABC/1

== system FOC_HF_G474/FOC/FOC_CURRENT/SVPWM/JudgeSector ==
  Valpha : Inport
  Vbeta : Inport  Port=2
  Constant : Constant  Value=0  OutDataTypeStr=single  SampleTime=-1
  If : If  IfExpression=u1
  If Action Subsystem : Subsystem  TreatAsAtomicUnit=on
  If Action Subsystem1 : Subsystem  TreatAsAtomicUnit=on
  Merge : Merge
  Relational Operator : RelationalOperator  OutDataTypeStr=boolean  RndMeth=Simplest
  Sector : Outport  OutMin=0  OutMax=6
  wires:
  Vbeta/1 -> Relational Operator/1, If Action Subsystem/2(Vbeta), If Action Subsystem1/2(Vbeta)
  If/1 -> If Action Subsystem/Action
  Valpha/1 -> If Action Subsystem1/1(Valpha), If Action Subsystem/1(Valpha)
  Merge/1 -> Sector/1
  If Action Subsystem/1(Sector) -> Merge/1
  If/2 -> If Action Subsystem1/Action
  If Action Subsystem1/1(Out1) -> Merge/2
  Relational Operator/1 -> If/1
  Constant/1 -> Relational Operator/2

== system FOC_HF_G474/FOC/FOC_CURRENT/InjectSolve/PLL/SpeedToTheta ==
  In1 : Inport
  RangeLimit : Subsystem
  Sum1 : Sum  Inputs=|++
  Ts : Gain  Gain=TsFOC
  Unit Delay : UnitDelay  SampleTime=-1  HasFrameUpgradeWarning=on
  Out1 : Outport
  wires:
  In1/1 -> Ts/1
  Ts/1 -> Sum1/1
  Sum1/1 -> RangeLimit/1(In)
  Unit Delay/1 -> Out1/1, Sum1/2
  RangeLimit/1(Theta) -> Unit Delay/1

== system FOC_HF_G474/FOC/FOC_CURRENT/InjectSolve/PLL/Subsystem ==
  In1 : Inport  OutDataTypeStr=double
  If : If  IfExpression=u1 > 0.78  ElseIfExpressions=u1 < -0.78
  If Action Subsystem : Subsystem  TreatAsAtomicUnit=on
  If Action Subsystem1 : Subsystem  TreatAsAtomicUnit=on
  If Action Subsystem2 : Subsystem  TreatAsAtomicUnit=on
  Merge : Merge  Inputs=3
  Output : Outport
  wires:
  In1/1 -> If Action Subsystem2/1(In1), If/1
  If/1 -> If Action Subsystem/Action
  If/2 -> If Action Subsystem1/Action
  If/3 -> If Action Subsystem2/Action
  If Action Subsystem/1(Out1) -> Merge/1
  If Action Subsystem1/1(Out1) -> Merge/2
  If Action Subsystem2/1(Out1) -> Merge/3
  Merge/1 -> Output/1

== system FOC_HF_G474/FOC/FOC_CURRENT/InjectSolve/QPLL/SpeedToTheta ==
  In1 : Inport
  RangeLimit : Subsystem
  Sum1 : Sum  Inputs=|++
  Ts : Gain  Gain=TsFOC
  Unit Delay : UnitDelay  SampleTime=-1  HasFrameUpgradeWarning=on
  Out1 : Outport
  wires:
  In1/1 -> Ts/1
  Ts/1 -> Sum1/1
  Sum1/1 -> RangeLimit/1(In)
  Unit Delay/1 -> Out1/1, Sum1/2
  RangeLimit/1(Theta) -> Unit Delay/1

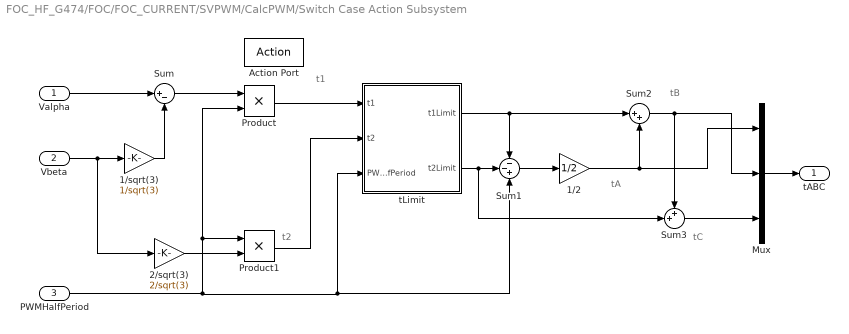
== system FOC_HF_G474/FOC/FOC_CURRENT/SVPWM/CalcPWM/Switch Case Action Subsystem ==
  note: tC
  note: tB
  note: tA
  note: t2
  note: t1
  Valpha : Inport
  Vbeta : Inport  Port=2
  PWMHalfPeriod : Inport  Port=3
  Action Port : ActionPort  ActionPortLabel=case [ 1 ]:
  1/2 : Gain  Gain=1/2
  1/sqrt(3) : Gain  Gain=1/sqrt(3)
  2/sqrt(3) : Gain  Gain=2/sqrt(3)
  Mux : Mux  Inputs=3
  Product : Product  OutMin=-1e4  OutMax=1e4
  Product1 : Product  OutMin=-1e4  OutMax=1e4
  Sum : Sum  Inputs=|+-  OutMin=-10  OutMax=10
  Sum1 : Sum  Inputs=--+  OutMin=-2e4  OutMax=2e4
  Sum2 : Sum  Inputs=|++  OutMin=-2e4  OutMax=2e4
  Sum3 : Sum  Inputs=++|  OutMin=-2e4  OutMax=2e4
  tLimit : Subsystem
  tABC : Outport
  wires:
  Valpha/1 -> Sum/1
  Vbeta/1 -> 2/sqrt(3)/1, 1/sqrt(3)/1
  1/sqrt(3)/1 -> Sum/2
  Sum/1 -> Product/1
  PWMHalfPeriod/1 -> Product/2, Product1/1, Sum1/3, tLimit/3(PWMHalfPeriod)
  2/sqrt(3)/1 -> Product1/2
  Sum1/1 -> 1/2/1
  1/2/1 -> Sum2/2, Mux/1
  Sum2/1 -> Mux/2, Sum3/1
  Sum3/1 -> Mux/3
  Mux/1 -> tABC/1
  Product/1 -> tLimit/1(t1)
  Product1/1 -> tLimit/2(t2)
  tLimit/1(t1Limit) -> Sum1/1, Sum2/1
  tLimit/2(t2Limit) -> Sum3/2, Sum1/2

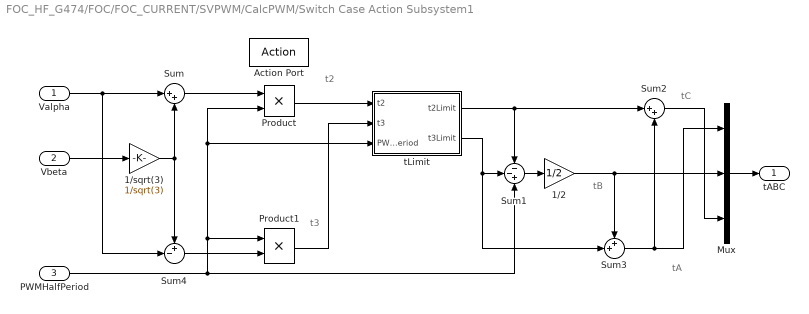
== system FOC_HF_G474/FOC/FOC_CURRENT/SVPWM/CalcPWM/Switch Case Action Subsystem1 ==
  note: tA
  note: tC
  note: tB
  note: t3
  note: t2
  Valpha : Inport
  Vbeta : Inport  Port=2
  PWMHalfPeriod : Inport  Port=3
  Action Port : ActionPort  ActionPortLabel=case [ 2 ]:
  1/2 : Gain  Gain=1/2
  1/sqrt(3) : Gain  Gain=1/sqrt(3)
  Mux : Mux  Inputs=3
  Product : Product  OutMin=-1e4  OutMax=1e4
  Product1 : Product  OutMin=-1e4  OutMax=1e4
  Sum : Sum  Inputs=|++  OutMin=-10  OutMax=10
  Sum1 : Sum  Inputs=--+  OutMin=-2e4  OutMax=2e4
  Sum2 : Sum  Inputs=|++  OutMin=-2e4  OutMax=2e4
  Sum3 : Sum  Inputs=++|  OutMin=-2e4  OutMax=2e4
  Sum4 : Sum  Inputs=+-|  OutMin=-10  OutMax=10
  tLimit : Subsystem
  tABC : Outport
  wires:
  Sum/1 -> Product/1
  Sum4/1 -> Product1/2
  PWMHalfPeriod/1 -> Sum1/3, tLimit/3(PWMHalfPeriod), Product/2, Product1/1
  1/2/1 -> Mux/2, Sum3/1
  Sum1/1 -> 1/2/1
  Sum2/1 -> Mux/3
  Sum3/1 -> Sum2/2, Mux/1
  Vbeta/1 -> 1/sqrt(3)/1
  1/sqrt(3)/1 -> Sum4/1, Sum/2
  Valpha/1 -> Sum4/2, Sum/1
  Mux/1 -> tABC/1
  Product/1 -> tLimit/1(t2)
  Product1/1 -> tLimit/2(t3)
  tLimit/1(t2Limit) -> Sum2/1, Sum1/1
  tLimit/2(t3Limit) -> Sum1/2, Sum3/2

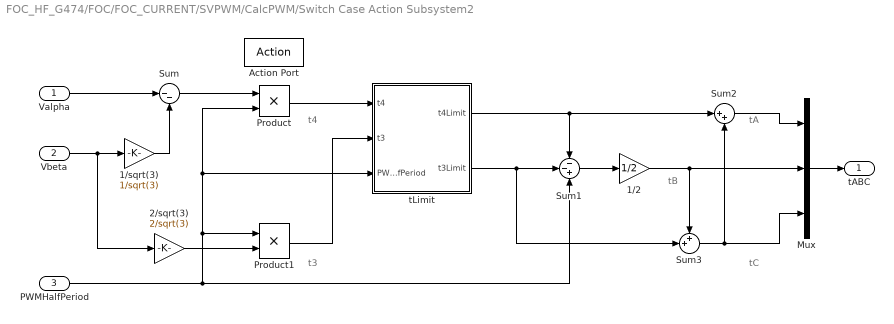
== system FOC_HF_G474/FOC/FOC_CURRENT/SVPWM/CalcPWM/Switch Case Action Subsystem2 ==
  note: tB
  note: tA
  note: t3
  note: t4
  note: tC
  Valpha : Inport
  Vbeta : Inport  Port=2
  PWMHalfPeriod : Inport  Port=3
  Action Port : ActionPort  ActionPortLabel=case [ 3 ]:
  1/2 : Gain  Gain=1/2
  1/sqrt(3) : Gain  Gain=1/sqrt(3)
  2/sqrt(3) : Gain  Gain=2/sqrt(3)
  Mux : Mux  Inputs=3
  Product : Product  OutMin=-1e4  OutMax=1e4
  Product1 : Product  OutMin=-1e4  OutMax=1e4
  Sum : Sum  Inputs=|--  OutMin=-10  OutMax=10
  Sum1 : Sum  Inputs=--+  OutMin=-2e4  OutMax=2e4
  Sum2 : Sum  Inputs=|++  OutMin=-2e4  OutMax=2e4
  Sum3 : Sum  Inputs=++|  OutMin=-2e4  OutMax=2e4
  tLimit : Subsystem
  tABC : Outport
  wires:
  Sum1/1 -> 1/2/1
  1/2/1 -> Mux/2, Sum3/1
  Vbeta/1 -> 2/sqrt(3)/1, 1/sqrt(3)/1
  2/sqrt(3)/1 -> Product1/2
  1/sqrt(3)/1 -> Sum/2
  Valpha/1 -> Sum/1
  Sum/1 -> Product/1
  Sum2/1 -> Mux/1
  PWMHalfPeriod/1 -> tLimit/3(PWMHalfPeriod), Product/2, Product1/1, Sum1/3
  Sum3/1 -> Sum2/2, Mux/3
  Mux/1 -> tABC/1
  Product/1 -> tLimit/1(t4)
  Product1/1 -> tLimit/2(t3)
  tLimit/1(t4Limit) -> Sum1/1, Sum2/1
  tLimit/2(t3Limit) -> Sum3/2, Sum1/2

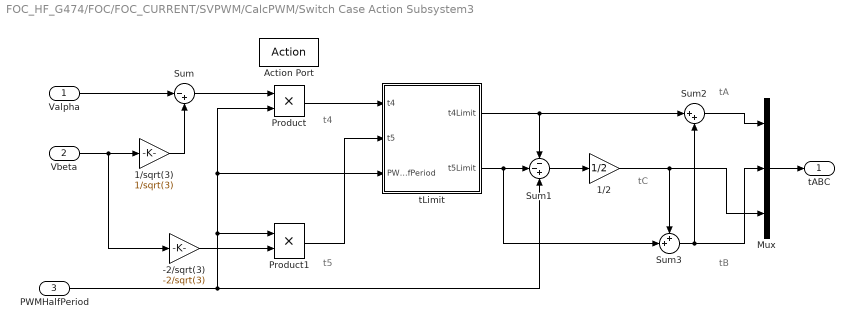
== system FOC_HF_G474/FOC/FOC_CURRENT/SVPWM/CalcPWM/Switch Case Action Subsystem3 ==
  note: tC
  note: tA
  note: t5
  note: t4
  note: tB
  Valpha : Inport
  Vbeta : Inport  Port=2
  PWMHalfPeriod : Inport  Port=3
  Action Port : ActionPort  ActionPortLabel=case [ 4 ]:
  -2/sqrt(3) : Gain  Gain=-2/sqrt(3)
  1/2 : Gain  Gain=1/2
  1/sqrt(3) : Gain  Gain=1/sqrt(3)
  Mux : Mux  Inputs=3
  Product : Product  OutMin=-1e4  OutMax=1e5
  Product1 : Product  OutMin=-1e4  OutMax=1e4
  Sum : Sum  Inputs=|-+  OutMin=-10  OutMax=10
  Sum1 : Sum  Inputs=--+  OutMin=-2e4  OutMax=2e4
  Sum2 : Sum  Inputs=|++  OutMin=-2e4  OutMax=2e4
  Sum3 : Sum  Inputs=++|  OutMin=-2e4  OutMax=2e4
  tLimit : Subsystem
  tABC : Outport
  wires:
  Sum1/1 -> 1/2/1
  1/2/1 -> Sum3/1, Mux/3
  Vbeta/1 -> -2/sqrt(3)/1, 1/sqrt(3)/1
  1/sqrt(3)/1 -> Sum/2
  Valpha/1 -> Sum/1
  Sum/1 -> Product/1
  Sum2/1 -> Mux/1
  PWMHalfPeriod/1 -> Sum1/3, tLimit/3(PWMHalfPeriod), Product/2, Product1/1
  Sum3/1 -> Sum2/2, Mux/2
  -2/sqrt(3)/1 -> Product1/2
  Mux/1 -> tABC/1
  Product/1 -> tLimit/1(t4)
  Product1/1 -> tLimit/2(t5)
  tLimit/2(t5Limit) -> Sum3/2, Sum1/2
  tLimit/1(t4Limit) -> Sum1/1, Sum2/1

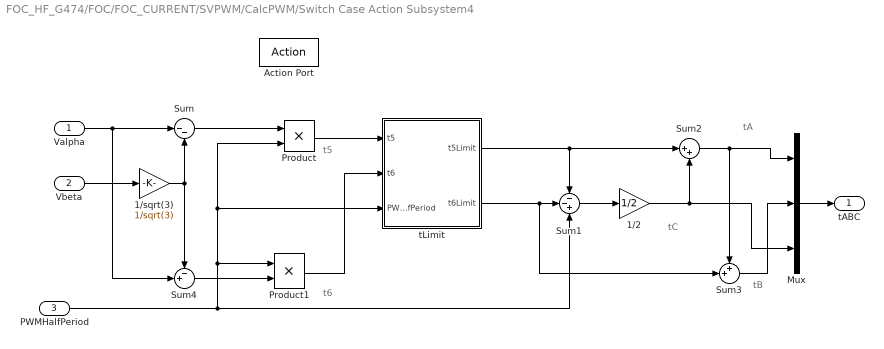
== system FOC_HF_G474/FOC/FOC_CURRENT/SVPWM/CalcPWM/Switch Case Action Subsystem4 ==
  note: tC
  note: tA
  note: t6
  note: t5
  note: tB
  Valpha : Inport
  Vbeta : Inport  Port=2
  PWMHalfPeriod : Inport  Port=3
  Action Port : ActionPort  ActionPortLabel=case [ 5 ]:
  1/2 : Gain  Gain=1/2
  1/sqrt(3) : Gain  Gain=1/sqrt(3)
  Mux : Mux  Inputs=3
  Product : Product  OutMin=-1e4  OutMax=1e4
  Product1 : Product  OutMin=-1e4  OutMax=1e4
  Sum : Sum  Inputs=|--  OutMin=-10  OutMax=10
  Sum1 : Sum  Inputs=--+  OutMin=-2e4  OutMax=2e4
  Sum2 : Sum  Inputs=|++  OutMin=-2e4  OutMax=2e4
  Sum3 : Sum  Inputs=++|  OutMin=-2e4  OutMax=2e4
  Sum4 : Sum  Inputs=-+|  OutMin=-10  OutMax=10
  tLimit : Subsystem
  tABC : Outport
  wires:
  Sum1/1 -> 1/2/1
  1/2/1 -> Mux/3, Sum2/2
  Vbeta/1 -> 1/sqrt(3)/1
  Sum4/1 -> Product1/2
  1/sqrt(3)/1 -> Sum/2, Sum4/1
  Valpha/1 -> Sum4/2, Sum/1
  Sum/1 -> Product/1
  Sum2/1 -> Mux/1, Sum3/1
  PWMHalfPeriod/1 -> tLimit/3(PWMHalfPeriod), Product/2, Product1/1, Sum1/3
  Sum3/1 -> Mux/2
  Mux/1 -> tABC/1
  Product/1 -> tLimit/1(t5)
  Product1/1 -> tLimit/2(t6)
  tLimit/2(t6Limit) -> Sum3/2, Sum1/2
  tLimit/1(t5Limit) -> Sum1/1, Sum2/1

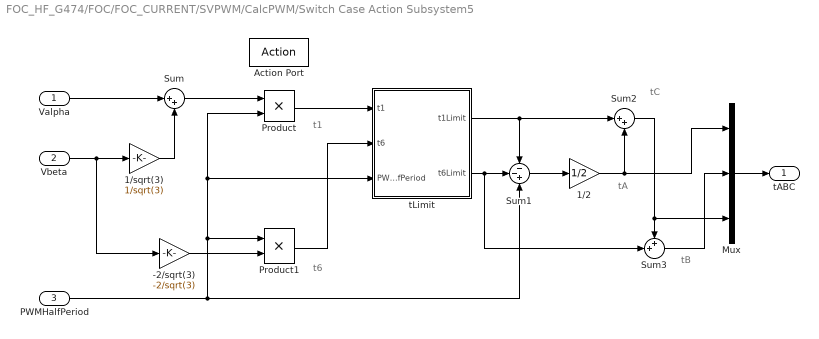
== system FOC_HF_G474/FOC/FOC_CURRENT/SVPWM/CalcPWM/Switch Case Action Subsystem5 ==
  note: tA
  note: tC
  note: t6
  note: t1
  note: tB
  Valpha : Inport
  Vbeta : Inport  Port=2
  PWMHalfPeriod : Inport  Port=3
  Action Port : ActionPort  ActionPortLabel=case [ 6 ]:
  -2/sqrt(3) : Gain  Gain=-2/sqrt(3)
  1/2 : Gain  Gain=1/2
  1/sqrt(3) : Gain  Gain=1/sqrt(3)
  Mux : Mux  Inputs=3
  Product : Product  OutMin=-1e4  OutMax=1e4
  Product1 : Product  OutMin=-1e4  OutMax=1e4
  Sum : Sum  Inputs=|++  OutMin=-10  OutMax=10
  Sum1 : Sum  Inputs=--+  OutMin=-2e4  OutMax=2e4
  Sum2 : Sum  Inputs=|++  OutMin=-2e4  OutMax=2e4
  Sum3 : Sum  Inputs=++|  OutMin=-2e4  OutMax=2E4
  tLimit : Subsystem
  tABC : Outport
  wires:
  Sum1/1 -> 1/2/1
  1/2/1 -> Mux/1, Sum2/2
  Vbeta/1 -> -2/sqrt(3)/1, 1/sqrt(3)/1
  1/sqrt(3)/1 -> Sum/2
  Valpha/1 -> Sum/1
  Sum/1 -> Product/1
  Sum2/1 -> Mux/3, Sum3/1
  Sum3/1 -> Mux/2
  -2/sqrt(3)/1 -> Product1/2
  Mux/1 -> tABC/1
  Product/1 -> tLimit/1(t1)
  Product1/1 -> tLimit/2(t6)
  PWMHalfPeriod/1 -> Sum1/3, Product/2, tLimit/3(PWMHalfPeriod), Product1/1
  tLimit/1(t1Limit) -> Sum1/1, Sum2/1
  tLimit/2(t6Limit) -> Sum3/2, Sum1/2

== system FOC_HF_G474/FOC/FOC_CURRENT/SVPWM/JudgeSector/If Action Subsystem ==
  Valpha : Inport
  Vbeta : Inport  Port=2
  Action Port : ActionPort  ActionPortLabel=if(u1)
  Constant : Constant  Value=0  OutDataTypeStr=single  SampleTime=-1
  If : If  IfExpression=u1
  If Action Subsystem : Subsystem  TreatAsAtomicUnit=on
  If Action Subsystem1 : Subsystem  TreatAsAtomicUnit=on
  Merge : Merge
  Relational Operator : RelationalOperator  OutDataTypeStr=boolean  RndMeth=Simplest
  Sector : Outport
  wires:
  Vbeta/1 -> If Action Subsystem/2(Vbeta), If Action Subsystem1/2(Vbeta)
  If/1 -> If Action Subsystem/Action
  If/2 -> If Action Subsystem1/Action
  If Action Subsystem/1(Sector) -> Merge/1
  If Action Subsystem1/1(Sector) -> Merge/2
  Merge/1 -> Sector/1
  Valpha/1 -> Relational Operator/1, If Action Subsystem/1(Valpha), If Action Subsystem1/1(Valpha)
  Relational Operator/1 -> If/1
  Constant/1 -> Relational Operator/2

== system FOC_HF_G474/FOC/FOC_CURRENT/SVPWM/JudgeSector/If Action Subsystem1 ==
  Valpha : Inport
  Vbeta : Inport  Port=2
  Action Port : ActionPort  ActionPortLabel=else
  Constant : Constant  Value=0  OutDataTypeStr=single  SampleTime=-1
  If : If  IfExpression=u1
  If Action Subsystem : Subsystem  TreatAsAtomicUnit=on
  If Action Subsystem1 : Subsystem  TreatAsAtomicUnit=on
  Merge : Merge
  Relational Operator : RelationalOperator  OutDataTypeStr=boolean  RndMeth=Simplest
  Out1 : Outport
  wires:
  If Action Subsystem/1(Sector) -> Merge/1
  Merge/1 -> Out1/1
  If/2 -> If Action Subsystem1/Action
  If Action Subsystem1/1(Sector) -> Merge/2
  If/1 -> If Action Subsystem/Action
  Valpha/1 -> If Action Subsystem/1(Valpha), If Action Subsystem1/1(Valpha), Relational Operator/1
  Vbeta/1 -> If Action Subsystem/2(Vbeta), If Action Subsystem1/2(Vbeta)
  Constant/1 -> Relational Operator/2
  Relational Operator/1 -> If/1

== system FOC_HF_G474/FOC/FOC_CURRENT/InjectSolve/PLL/SpeedToTheta/RangeLimit ==
  In : Inport
  Constant : Constant  Value=pi  SampleTime=-1
  Constant1 : Constant  Value=-pi  SampleTime=-1
  If : If  NumInputs=2  IfExpression=u1  ElseIfExpressions=u2
  If Action Subsystem : Subsystem  TreatAsAtomicUnit=on
  If Action Subsystem1 : Subsystem  TreatAsAtomicUnit=on
  If Action Subsystem2 : Subsystem  TreatAsAtomicUnit=on
  Merge : Merge  Inputs=3
  Relational Operator : RelationalOperator  Operator=>  OutDataTypeStr=boolean  RndMeth=Simplest
  Relational Operator1 : RelationalOperator  Operator=<  OutDataTypeStr=boolean  RndMeth=Simplest
  Theta : Outport  OutMin=-pi  OutMax=pi
  wires:
  Relational Operator/1 -> If/1
  Constant/1 -> Relational Operator/2
  Constant1/1 -> Relational Operator1/2
  In/1 -> Relational Operator1/1, If Action Subsystem2/1(In1), If Action Subsystem1/1(In1), If Action Subsystem/1(In1), Relational Operator/1
  Relational Operator1/1 -> If/2
  Merge/1 -> Theta/1
  If/3 -> If Action Subsystem2/Action
  If/2 -> If Action Subsystem/Action
  If/1 -> If Action Subsystem1/Action
  If Action Subsystem2/1(Out1) -> Merge/1
  If Action Subsystem/1(Out1) -> Merge/2
  If Action Subsystem1/1(Out1) -> Merge/3

== system FOC_HF_G474/FOC/FOC_CURRENT/InjectSolve/PLL/Subsystem/If Action Subsystem ==
  Action Port : ActionPort
  Constant : Constant  Value=0  SampleTime=-1
  Out1 : Outport
  wires:
  Constant/1 -> Out1/1

== system FOC_HF_G474/FOC/FOC_CURRENT/InjectSolve/PLL/Subsystem/If Action Subsystem1 ==
  Action Port : ActionPort
  Constant : Constant  Value=0  SampleTime=-1
  Out1 : Outport
  wires:
  Constant/1 -> Out1/1

== system FOC_HF_G474/FOC/FOC_CURRENT/InjectSolve/PLL/Subsystem/If Action Subsystem2 ==
  In1 : Inport
  Action Port : ActionPort
  Out1 : Outport  OutDataTypeStr=double
  wires:
  In1/1 -> Out1/1

== system FOC_HF_G474/FOC/FOC_CURRENT/InjectSolve/QPLL/SpeedToTheta/RangeLimit ==
  In : Inport
  Constant : Constant  Value=2*pi  OutDataTypeStr=single  SampleTime=-1
  Constant1 : Constant  Value=0  OutDataTypeStr=single  SampleTime=-1
  If : If  NumInputs=2  IfExpression=u1  ElseIfExpressions=u2
  If Action Subsystem : Subsystem  TreatAsAtomicUnit=on
  If Action Subsystem1 : Subsystem  TreatAsAtomicUnit=on
  If Action Subsystem2 : Subsystem  TreatAsAtomicUnit=on
  Merge : Merge  Inputs=3
  Relational Operator : RelationalOperator  Operator=>  OutDataTypeStr=boolean  RndMeth=Simplest
  Relational Operator1 : RelationalOperator  Operator=<  OutDataTypeStr=boolean  RndMeth=Simplest
  Theta : Outport
  wires:
  Relational Operator/1 -> If/1
  Constant/1 -> Relational Operator/2
  Constant1/1 -> Relational Operator1/2
  In/1 -> Relational Operator1/1, If Action Subsystem2/1(In1), If Action Subsystem1/1(In1), If Action Subsystem/1(In1), Relational Operator/1
  Relational Operator1/1 -> If/2
  Merge/1 -> Theta/1
  If/3 -> If Action Subsystem2/Action
  If/2 -> If Action Subsystem/Action
  If/1 -> If Action Subsystem1/Action
  If Action Subsystem2/1(Out1) -> Merge/1
  If Action Subsystem/1(Out1) -> Merge/2
  If Action Subsystem1/1(Out1) -> Merge/3
